simulink model "upravljacFinal"  (R2019b)
settings: Solver=FixedStepAuto  StartTime=0.0  StopTime=1000  FixedStep=0.1  RelTol=1e-3
libraries: fuzblock x1
settings Model: Creator=Kosta  LastModifiedBy=Kosta

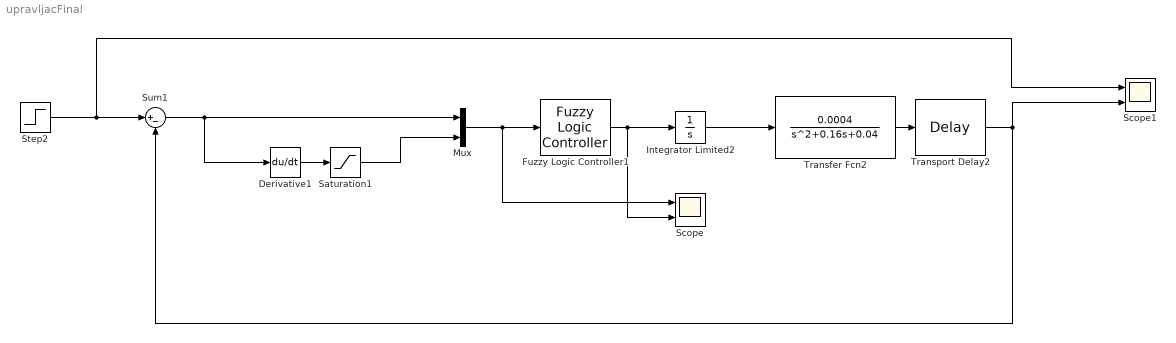
== system upravljacFinal ==
  Derivative1 : Derivative
  Fuzzy Logic Controller1 : fuzblock/Fuzzy Logic  Controller  FIS='upravljacf4final.fis'  OutputSampleNumber=101  DataType=double  FuzzifiedInputs=off  RuleFiringStrengths=off  RuleOutputs=off  AggregatedOutputs=off  SimulateUsing=Interpreted execution  OutOfRangeInputValueMessage=warning  NoRuleFiredMessage=warning  EmptyOutputFuzzySetMessage=warning
  Integrator Limited2 : Integrator  LimitOutput=on  UpperSaturationLimit=50  LowerSaturationLimit=-50
  Mux : Mux  Inputs=2
  Saturation1 : Saturate  UpperLimit=0.025  LowerLimit=-0.025
  Scope : Scope  NumInputPorts=2
  Scope1 : Scope  NumInputPorts=2
  Step2 : Step  Time=500  Before=-0.4  After=0.4  SampleTime=0
  Sum1 : Sum  Inputs=|+-
  Transfer Fcn2 : TransferFcn  Numerator=[0.0004]  Denominator=[1 0.16 0.04]
  Transport Delay2 : TransportDelay  DelayTime=2
  wires:
  Transfer Fcn2/1 -> Transport Delay2/1
  Sum1/1 -> Mux/1, Derivative1/1
  Transport Delay2/1 -> Scope1/2, Sum1/2
  Mux/1 -> Scope/1, Fuzzy Logic Controller1/1
  Saturation1/1 -> Mux/2
  Step2/1 -> Scope1/1, Sum1/1
  Integrator Limited2/1 -> Transfer Fcn2/1
  Derivative1/1 -> Saturation1/1
  Fuzzy Logic Controller1/1 -> Scope/2, Integrator Limited2/1
